simulink model "Figure3"  (R2021b)
settings: Solver=VariableStepAuto  StartTime=0.0  StopTime=10.0  RelTol=1e-3
undefined symbols (not defined in the file or in its folder): get, gray, res
libraries: myLib_CustomBoolean x35, dspobslib x1
settings Model: Creator=matt  LastModifiedBy=matt

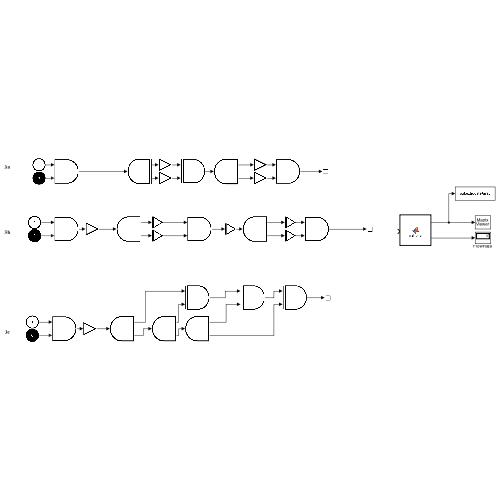
[thumbnail: Simulink's stored preview of the top-level diagram]
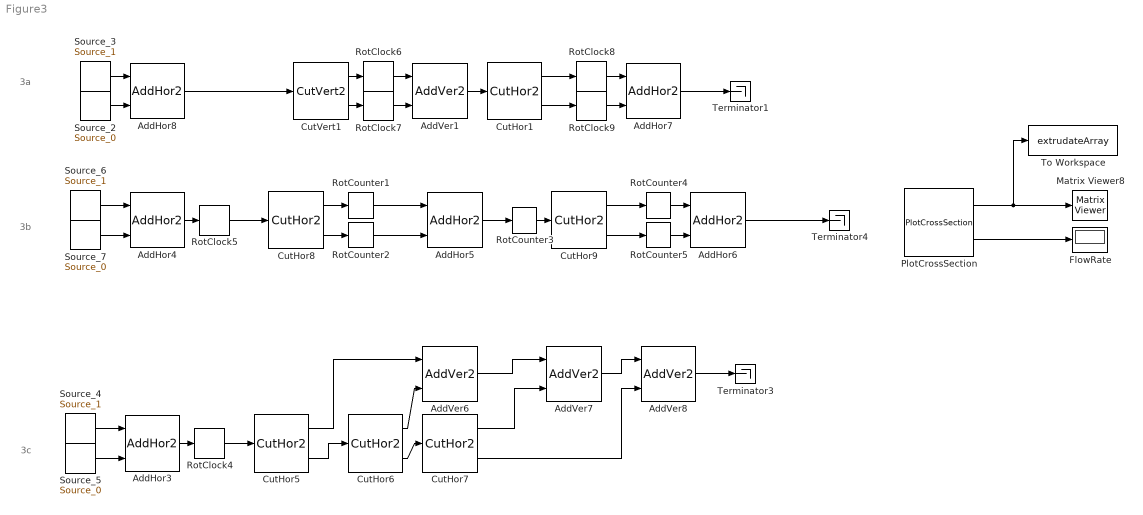
== system Figure3 ==
  note: 3a
  note: 3b
  note: 3c
  AddHor{3..8} (6 alike) : myLib_CustomBoolean/AddHor2  SystemSampleTime=-1  VariantActivationTime=update diagram  Latency=0  AutoFrameSizeCalculation=off
      settings: SourceProductName=Boolean_Custom_Library
  AddVer{1,6..8} (4 alike) : myLib_CustomBoolean/AddVer2  SystemSampleTime=-1  VariantActivationTime=update diagram  Latency=0  AutoFrameSizeCalculation=off
      settings: SourceProductName=Boolean_Custom_Library
  CutHor{1,5..9} (6 alike) : myLib_CustomBoolean/CutHor2  SystemSampleTime=-1  VariantActivationTime=update diagram  Latency=0  AutoFrameSizeCalculation=off
      settings: SourceProductName=Boolean_Custom_Library
  CutVert1 : myLib_CustomBoolean/CutVert2  SystemSampleTime=-1  VariantActivationTime=update diagram  Latency=0  AutoFrameSizeCalculation=off
      settings: SourceProductName=Boolean_Custom_Library
  FlowRate : Display
  Matrix Viewer8 : dspobslib/Matrix Viewer  ImageParams=off  CMapStr=gray(3)  AxisColorbar=on  AxisParams=off  AxisOrigin=Upper left corner  AxisTickMode=User-defined  XTickRange=[0 1]  YTickRange=[0 1]  XLabel=X-axis  YLabel=Y-axis  ZLabel=Z-axis  FigPos=get(0,'defaultfigureposition')  AxisZoom=off
      settings: SourceProductBaseCode=DS  YMin=0  YMax=1
  PlotCrossSection : myLib_CustomBoolean/PlotCrossSection  SystemSampleTime=-1  VariantActivationTime=update diagram  Latency=0  AutoFrameSizeCalculation=off
      settings: SourceProductName=Boolean_Custom_Library
  RotClock{4..9} (6 alike) : myLib_CustomBoolean/RotClock  SystemSampleTime=-1  VariantActivationTime=update diagram  Latency=0  AutoFrameSizeCalculation=off
      settings: SourceProductName=Boolean_Custom_Library
  RotCounter{1..5} (5 alike) : myLib_CustomBoolean/RotCounter  SystemSampleTime=-1  VariantActivationTime=update diagram  Latency=0  AutoFrameSizeCalculation=off
      settings: SourceProductName=Boolean_Custom_Library
  Source_2 : myLib_CustomBoolean/Source_0  Value=cat(3, 0.*ones(res,res), 1.0.*ones(res,res))  VectorParams1D=off  OutMin=[]  OutMax=[]  OutDataTypeStr=Inherit: Inherit from 'Constant value'  SampleTime=inf  FramePeriod=inf
      settings: SourceProductName=Boolean_Custom_Library
  Source_3 : myLib_CustomBoolean/Source_1  Value=cat(3, 1.*ones(res,res), 1.0*ones(res,res))  VectorParams1D=off  OutMin=[]  OutMax=[]  OutDataTypeStr=Inherit: Inherit from 'Constant value'  SampleTime=inf  FramePeriod=inf
      settings: SourceProductName=Boolean_Custom_Library
  Source_4 : myLib_CustomBoolean/Source_1  Value=cat(3, 1.*ones(res,res), 1.0*ones(res,res))  VectorParams1D=off  OutMin=[]  OutMax=[]  OutDataTypeStr=Inherit: Inherit from 'Constant value'  SampleTime=inf  FramePeriod=inf
      settings: SourceProductName=Boolean_Custom_Library
  Source_5 : myLib_CustomBoolean/Source_0  Value=cat(3, 0.*ones(res,res), 1.0.*ones(res,res))  VectorParams1D=off  OutMin=[]  OutMax=[]  OutDataTypeStr=Inherit: Inherit from 'Constant value'  SampleTime=inf  FramePeriod=inf
      settings: SourceProductName=Boolean_Custom_Library
  Source_6 : myLib_CustomBoolean/Source_1  Value=cat(3, 1.*ones(res,res), 1.0*ones(res,res))  VectorParams1D=off  OutMin=[]  OutMax=[]  OutDataTypeStr=Inherit: Inherit from 'Constant value'  SampleTime=inf  FramePeriod=inf
      settings: SourceProductName=Boolean_Custom_Library
  Source_7 : myLib_CustomBoolean/Source_0  Value=cat(3, 0.*ones(res,res), 1.0.*ones(res,res))  VectorParams1D=off  OutMin=[]  OutMax=[]  OutDataTypeStr=Inherit: Inherit from 'Constant value'  SampleTime=inf  FramePeriod=inf
      settings: SourceProductName=Boolean_Custom_Library
  Terminator1 : Terminator
  Terminator3 : Terminator
  Terminator4 : Terminator
  To Workspace : ToWorkspace  VariableName=extrudateArray  SampleTime=51
  wires:
  AddHor7/1 -> Terminator1/1
  AddHor8/1 -> CutVert1/1
  RotClock8/1 -> AddHor7/1
  RotClock7/1 -> AddVer1/2
  CutHor1/2 -> RotClock9/1
  Source_3/1 -> AddHor8/1
  CutVert1/2 -> RotClock7/1
  CutVert1/1 -> RotClock6/1
  AddVer1/1 -> CutHor1/1
  RotClock6/1 -> AddVer1/1
  CutHor1/1 -> RotClock8/1
  RotClock9/1 -> AddHor7/2
  Source_2/1 -> AddHor8/2
  AddHor5/1 -> RotCounter3/1
  CutHor8/1 -> RotCounter1/1
  Source_7/1 -> AddHor4/2
  RotCounter4/1 -> AddHor6/1
  Source_6/1 -> AddHor4/1
  RotCounter5/1 -> AddHor6/2
  RotClock5/1 -> CutHor8/1
  CutHor9/1 -> RotCounter4/1
  AddHor6/1 -> Terminator4/1
  RotCounter2/1 -> AddHor5/2
  CutHor8/2 -> RotCounter2/1
  RotCounter3/1 -> CutHor9/1
  AddHor4/1 -> RotClock5/1
  CutHor9/2 -> RotCounter5/1
  RotCounter1/1 -> AddHor5/1
  AddVer6/1 -> AddVer7/1
  CutHor6/2 -> CutHor7/1
  AddVer7/1 -> AddVer8/1
  AddVer8/1 -> Terminator3/1
  AddHor3/1 -> RotClock4/1
  CutHor7/1 -> AddVer7/2
  Source_5/1 -> AddHor3/2
  CutHor7/2 -> AddVer8/2
  Source_4/1 -> AddHor3/1
  CutHor6/1 -> AddVer6/2
  CutHor5/1 -> AddVer6/1
  RotClock4/1 -> CutHor5/1
  CutHor5/2 -> CutHor6/1
  PlotCrossSection/2 -> FlowRate/1
  PlotCrossSection/1 -> To Workspace/1, Matrix Viewer8/1
